simulink subsystem "PvtSubSys_VSM_ALL"  (R2020b)
settings: Solver=VariableStepAuto  StartTime=0.0  StopTime=10.0  RelTol=1e-3
values from neighbouring files (symbols this model uses):
  P_VSM_NOH_Act_Req = 0    [VSM_All.sldd]
  P_VSM_NOH_Swt_Req = 0    [VSM_All.sldd]
undefined symbols (not defined in the file or in its folder): ACC_STATE, HWA_STATE, LCK_STATE, P_VSM_ACCSOS_SW, P_VSM_AESSwtReq, P_VSM_CruiseFunUserInputMappingWays, P_VSM_ELKSwtReq, P_VSM_ESS_VehSwtReq, P_VSM_HWA_DMS_Enable, P_VSM_ICA_HandsOffSwtReq, P_VSM_IntelligentEvaSwtReq, P_VSM_ISLSwtReq, P_VSM_LCKSwtReq, P_VSM_LDWSwtReq, P_VSM_LKASwtReq, P_VSM_LSSSwtReq, P_VSM_PowerTrainConfig, P_VSM_SOSContinueTime, P_VSM_SOSSpdLimit, P_VSM_TSR_Dis_keep_SPL_Table, P_VSM_TSR_Dis_keep_SPLend, P_VSM_TSR_Dis_keep_TS_Table, P_VSM_TSR_Ena_SPLSupp_Table, P_VSM_TSR_Ena_TS_Table, P_VSM_TSR_SLIF_Speed_High, P_VSM_TSR_SLIF_Speed_Low, P_VSM_TSR_SLW_SnvtySwitch, P_VSM_TSR_SLW_Speed_Delta_disable, P_VSM_TSR_SLW_Speed_Delta_enable, P_VSM_TSR_SLW_Speed_High, P_VSM_TSR_SLW_Speed_Low, P_VSM_TSR_SLW_TrafEyeAvtiveDist, P_VSM_TSR_SLW_Warning_Time, P_VSM_TSR_SteerWheelAngle, P_VSM_TSR_SWS_speed_withDir, P_VSM_TSR_SWS_speed_woDir, P_VSM_TSRSwtReq, P_VSM_TSRWarnSwtReq, TJA_STATE, User_LC_ALCswt, User_LC_DrvConfirm, User_LC_DrvLCswt, User_LC_DrvOverride, User_LC_LeTurnNextLineReq, User_LC_RiTurnNextLineReq, User_LC_TurnMostLeLineReq, User_LC_TurnMostRiLineReq, User_LeTurnLmpOn, User_RiTurnLmpOn
libraries: simulink x51
(part 3 of 7)

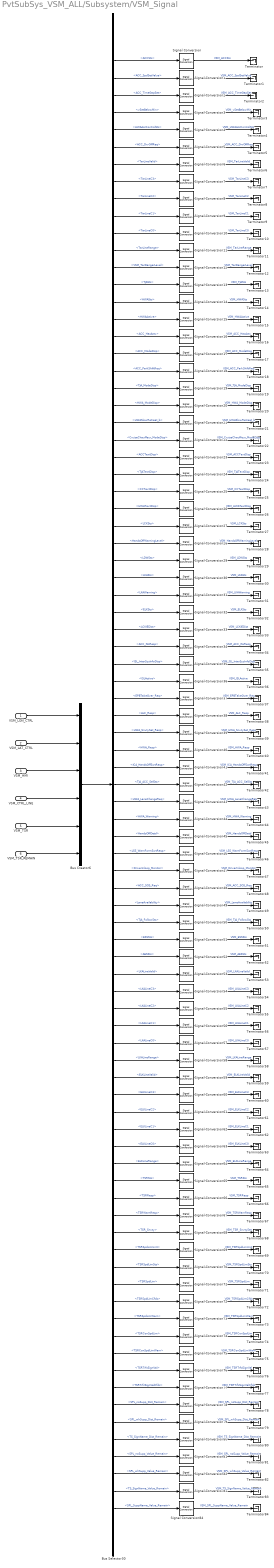
== system PvtSubSys_VSM_ALL/Subsystem/VSM_Signal ==
  VSM_LON_CTRL : Inport
  VSM_LAT_CTRL : Inport  Port=2
  VSM_HMI : Inport  Port=3
  VSM_CTRL_LINE : Inport  Port=4
  VSM_TSR : Inport  Port=5
  VSM_TSR_REMAIN : Inport  Port=6
  Bus Creator6 : BusCreator  Inputs=6
  Bus Selector30 : BusSelector  OutputSignals=VSM_LON_CTRL.ACCSts,VSM_LON_CTRL.ACC_SpdSetValue,VSM_LON_CTRL.ACC_TimeGapSet,VSM_LON_CTRL.vSetBelowMin,VSM_LON_CTRL.HWAAccControlSts,VSM_LON_CTRL.ACC_DrvOffReq,VSM_LAT_CTRL.TarLineValid,VSM_LAT_CTRL.TarLineC3,VSM_LAT_CTRL.TarLineC2,VSM_LAT_CTRL.TarLineC1,VSM_LAT_CTRL.TarLineC0,VSM_LAT_CTRL.TarLineRange,VSM_LAT_CTRL.VSM_TarDangerLevel,VSM_HMI.TJASts,VSM_HMI.HWASts,VSM_HMI.HWAActive,VSM_HMI.ACC_HazActv,VSM_HMI.ACC_ModeDisp,VSM_HMI.ACC_ParkShiftReq,VSM_HMI.TJA_ModeDisp,VSM_HMI.HWA_ModeDisp,VSM_HMI.HWASlowRetreat_b,VSM_HMI.CruiseChauffeur_ModeDisp,VSM_HMI.ACCTextDisp,VSM_HMI.TJATextDisp,VSM_HMI.CCTextDisp,VSM_HMI.HWATextDisp,VSM_HMI.LCKSts,VSM_HMI.HandsOffWarningLevel,VSM_HMI.LDWSts,VSM_HMI.LKASts,VSM_HMI.LKAWarning,VSM_HMI.ELKSts,VSM_HMI.LCKIEDist,VSM_HMI.ACC_ISLResp,VSM_HMI.ISL_InterSysInfoDisp,VSM_HMI.ISLActive,VSM_HMI.EPBTakeOver_Req,VSM_HMI.ALC_Resp,VSM_HMI.HWA_SnvtySet_Resp,VSM_HMI.HWA_Resp,VSM_HMI.ICA_HandsOffSwtResp,VSM_HMI.TJA_ACC_SelSts,VSM_HMI.HWA_LaneChangeReq,VSM_HMI.HWA_Warning,VSM_HMI.HandsOffDetd,VSM_HMI.LSS_WarnFormSwtResp,VSM_HMI.DriverInloop_Monitor,VSM_HMI.ACC_SOS_Req,VSM_HMI.LaneAvailability,VSM_HMI.TJA_FollowSts,VSM_HMI.ESSSts,VSM_HMI.AESSts,VSM_CTRL_LINE.LKALineValid,VSM_CTRL_LINE.LKALineC3,VSM_CTRL_LINE.LKALineC2,VSM_CTRL_LINE.LKALineC1,VSM_CTRL_LINE.LKALineC0,VSM_CTRL_LINE.LKALineRange,VSM_CTRL_LINE.ELKLineValid,VSM_CTRL_LINE.ELKLineC3,VSM_CTRL_LINE.ELKLineC2,VSM_CTRL_LINE.ELKLineC1,VSM_CTRL_LINE.ELKLineC0,VSM_CTRL_LINE.ELKLineRange,VSM_TSR.TSRSts,VSM_TSR.TSRResp,VSM_TSR.TSRWarnResp,VSM_TSR.TSR_Snvty,VSM_TSR.TSRSpdLimUnit,VSM_TSR.TSRSpdLimSts,VSM_TSR.TSRSpdLim,VSM_TSR.TSRSpdLimCfdc,VSM_TSR.TSRSpdLimWarn,VSM_TSR.TSRConSpdLim,VSM_TSR.TSRConSpdLimWarn,VSM_TSR.TSRTrfcSignVal,VSM_TSR.TSRTrfcSignValCfdc,VSM_TSR_REMAIN.SPL_noSupp_Dist_Remain,VSM_TSR_REMAIN.SPL_whSupp_Dist_Remain,VSM_TSR_REMAIN.TS_SignName_Dist_Remain,VSM_TSR_REMAIN.SPL_noSupp_Value_Remain,VSM_TSR_REMAIN.SPL_whSupp_Value_Remain,VSM_TSR_REMAIN.TS_SignName_Value_Remain,VSM_TSR_REMAIN.SPL_SuppName_Value_Remain
  Signal Conversion{,1..84} (85 alike) : SignalConversion  OverrideOpt=off
  Terminator{,1..84} (85 alike) : Terminator
  wires:
  Signal Conversion84/1 -> Terminator84/1  "VSM_SPL_SuppName_Value_Remain"
  Bus Selector30/85 -> Signal Conversion84/1  "<SPL_SuppName_Value_Remain>"
  Bus Selector30/84 -> Signal Conversion83/1  "<TS_SignName_Value_Remain>"
  Signal Conversion83/1 -> Terminator83/1  "VSM_TS_SignName_Value_Remain"
  Signal Conversion82/1 -> Terminator82/1  "VSM_SPL_whSupp_Value_Remain"
  Bus Selector30/83 -> Signal Conversion82/1  "<SPL_whSupp_Value_Remain>"
  Bus Selector30/82 -> Signal Conversion81/1  "<SPL_noSupp_Value_Remain>"
  Signal Conversion81/1 -> Terminator81/1  "VSM_SPL_noSupp_Value_Remain"
  Signal Conversion80/1 -> Terminator80/1  "VSM_TS_SignName_Dist_Remain"
  Bus Selector30/81 -> Signal Conversion80/1  "<TS_SignName_Dist_Remain>"
  Bus Selector30/80 -> Signal Conversion79/1  "<SPL_whSupp_Dist_Remain>"
  Signal Conversion79/1 -> Terminator79/1  "VSM_SPL_whSupp_Dist_Remain"
  Signal Conversion78/1 -> Terminator78/1  "VSM_SPL_noSupp_Dist_Remain"
  Bus Selector30/79 -> Signal Conversion78/1  "<SPL_noSupp_Dist_Remain>"
  Bus Selector30/78 -> Signal Conversion77/1  "<TSRTrfcSignValCfdc>"
  Signal Conversion77/1 -> Terminator77/1  "VSM_TSRTrfcSignValCfdc"
  Signal Conversion76/1 -> Terminator76/1  "VSM_TSRTrfcSignVal"
  Bus Selector30/77 -> Signal Conversion76/1  "<TSRTrfcSignVal>"
  Bus Selector30/76 -> Signal Conversion75/1  "<TSRConSpdLimWarn>"
  Signal Conversion75/1 -> Terminator75/1  "VSM_TSRConSpdLimWarn"
  Signal Conversion74/1 -> Terminator74/1  "VSM_TSRConSpdLim"
  Bus Selector30/75 -> Signal Conversion74/1  "<TSRConSpdLim>"
  Bus Selector30/74 -> Signal Conversion73/1  "<TSRSpdLimWarn>"
  Signal Conversion73/1 -> Terminator73/1  "VSM_TSRSpdLimWarn"
  Signal Conversion72/1 -> Terminator72/1  "VSM_TSRSpdLimCfdc"
  Bus Selector30/73 -> Signal Conversion72/1  "<TSRSpdLimCfdc>"
  Bus Selector30/72 -> Signal Conversion71/1  "<TSRSpdLim>"
  Signal Conversion71/1 -> Terminator71/1  "VSM_TSRSpdLim"
  Signal Conversion70/1 -> Terminator70/1  "VSM_TSRSpdLimSts"
  Bus Selector30/71 -> Signal Conversion70/1  "<TSRSpdLimSts>"
  Bus Selector30/70 -> Signal Conversion69/1  "<TSRSpdLimUnit>"
  Signal Conversion69/1 -> Terminator69/1  "VSM_TSRSpdLimUnit"
  Signal Conversion68/1 -> Terminator68/1  "VSM_TSR_SnvtySet"
  Bus Selector30/69 -> Signal Conversion68/1  "<TSR_Snvty>"
  Bus Selector30/68 -> Signal Conversion67/1  "<TSRWarnResp>"
  Signal Conversion67/1 -> Terminator67/1  "VSM_TSRWarnResp"
  Signal Conversion66/1 -> Terminator66/1  "VSM_TSRResp"
  Bus Selector30/67 -> Signal Conversion66/1  "<TSRResp>"
  Bus Selector30/66 -> Signal Conversion65/1  "<TSRSts>"
  Signal Conversion65/1 -> Terminator65/1  "VSM_TSRSts"
  Signal Conversion64/1 -> Terminator64/1  "VSM_ELKLineRange"
  Bus Selector30/65 -> Signal Conversion64/1  "<ELKLineRange>"
  Bus Selector30/64 -> Signal Conversion63/1  "<ELKLineC0>"
  Signal Conversion63/1 -> Terminator63/1  "VSM_ELKLineC0"
  Signal Conversion62/1 -> Terminator62/1  "VSM_ELKLineC1"
  Bus Selector30/63 -> Signal Conversion62/1  "<ELKLineC1>"
  Bus Selector30/62 -> Signal Conversion61/1  "<ELKLineC2>"
  Signal Conversion61/1 -> Terminator61/1  "VSM_ELKLineC2"
  Signal Conversion60/1 -> Terminator60/1  "VSM_ELKLineC3"
  Bus Selector30/61 -> Signal Conversion60/1  "<ELKLineC3>"
  Bus Selector30/60 -> Signal Conversion59/1  "<ELKLineValid>"
  Signal Conversion59/1 -> Terminator59/1  "VSM_ELKLineValid"
  Signal Conversion58/1 -> Terminator58/1  "VSM_LKALineRange"
  Bus Selector30/59 -> Signal Conversion58/1  "<LKALineRange>"
  Bus Selector30/58 -> Signal Conversion57/1  "<LKALineC0>"
  Signal Conversion57/1 -> Terminator57/1  "VSM_LKALineC0"
  Signal Conversion56/1 -> Terminator56/1  "VSM_LKALineC1"
  Bus Selector30/57 -> Signal Conversion56/1  "<LKALineC1>"
  Bus Selector30/56 -> Signal Conversion55/1  "<LKALineC2>"
  Signal Conversion55/1 -> Terminator55/1  "VSM_LKALineC2"
  Signal Conversion54/1 -> Terminator54/1  "VSM_LKALineC3"
  Bus Selector30/55 -> Signal Conversion54/1  "<LKALineC3>"
  Bus Selector30/54 -> Signal Conversion53/1  "<LKALineValid>"
  Signal Conversion53/1 -> Terminator53/1  "VSM_LKALineValid"
  Signal Conversion52/1 -> Terminator52/1  "VSM_AESSts"
  Bus Selector30/53 -> Signal Conversion52/1  "<AESSts>"
  Bus Selector30/52 -> Signal Conversion51/1  "<ESSSts>"
  Signal Conversion51/1 -> Terminator51/1  "VSM_ESSSts"
  Signal Conversion50/1 -> Terminator50/1  "VSM_TJA_FollowSts"
  Bus Selector30/51 -> Signal Conversion50/1  "<TJA_FollowSts>"
  Bus Selector30/50 -> Signal Conversion49/1  "<LaneAvailability>"
  Signal Conversion49/1 -> Terminator49/1  "VSM_LaneAvailability"
  Signal Conversion48/1 -> Terminator48/1  "VSM_ACC_SOS_Req"
  Bus Selector30/49 -> Signal Conversion48/1  "<ACC_SOS_Req>"
  Bus Selector30/48 -> Signal Conversion47/1  "<DriverInloop_Monitor>"
  Signal Conversion47/1 -> Terminator47/1  "VSM_DriverInloop_Monitor"
  Signal Conversion46/1 -> Terminator46/1  "VSM_LSS_WarnFormSwtResp"
  Bus Selector30/47 -> Signal Conversion46/1  "<LSS_WarnFormSwtResp>"
  Bus Selector30/46 -> Signal Conversion45/1  "<HandsOffDetd>"
  Signal Conversion45/1 -> Terminator45/1  "VSM_HandsOffDetd"
  Signal Conversion44/1 -> Terminator44/1  "VSM_HWA_Warning"
  Bus Selector30/45 -> Signal Conversion44/1  "<HWA_Warning>"
  Bus Selector30/44 -> Signal Conversion43/1  "<HWA_LaneChangeReq>"
  Signal Conversion43/1 -> Terminator43/1  "VSM_HWA_LaneChangeReq"
  Signal Conversion42/1 -> Terminator42/1  "VSM_TJA_ACC_SelSts"
  Bus Selector30/43 -> Signal Conversion42/1  "<TJA_ACC_SelSts>"
  Bus Selector30/42 -> Signal Conversion41/1  "<ICA_HandsOffSwtResp>"
  Signal Conversion41/1 -> Terminator41/1  "VSM_ICA_HandsOffSwtResp"
  Signal Conversion40/1 -> Terminator40/1  "VSM_HWA_Resp"
  Bus Selector30/41 -> Signal Conversion40/1  "<HWA_Resp>"
  Bus Selector30/40 -> Signal Conversion39/1  "<HWA_SnvtySet_Resp>"
  Signal Conversion39/1 -> Terminator39/1  "VSM_HWA_SnvtySet_Resp"
  Signal Conversion38/1 -> Terminator38/1  "VSM_ALC_Resp"
  Bus Selector30/39 -> Signal Conversion38/1  "<ALC_Resp>"
  Bus Selector30/38 -> Signal Conversion37/1  "<EPBTakeOver_Req>"
  Signal Conversion37/1 -> Terminator37/1  "VSM_EPBTakeOver_Req"
  Signal Conversion36/1 -> Terminator36/1  "VSM_ISLActive"
  Bus Selector30/37 -> Signal Conversion36/1  "<ISLActive>"
  Bus Selector30/36 -> Signal Conversion35/1  "<ISL_InterSysInfoDisp>"
  Signal Conversion35/1 -> Terminator35/1  "VSM_ISL_InterSysInfoDisp"
  Signal Conversion34/1 -> Terminator34/1  "VSM_ACC_ISLResp"
  Bus Selector30/35 -> Signal Conversion34/1  "<ACC_ISLResp>"
  Bus Selector30/34 -> Signal Conversion33/1  "<LCKIEDist>"
  Signal Conversion33/1 -> Terminator33/1  "VSM_LCKIEDist"
  Signal Conversion32/1 -> Terminator32/1  "VSM_ELKSts"
  Bus Selector30/33 -> Signal Conversion32/1  "<ELKSts>"
  Bus Selector30/32 -> Signal Conversion31/1  "<LKAWarning>"
  Signal Conversion31/1 -> Terminator31/1  "VSM_LKAWarning"
  Signal Conversion30/1 -> Terminator30/1  "VSM_LKASts"
  Bus Selector30/31 -> Signal Conversion30/1  "<LKASts>"
  Bus Selector30/30 -> Signal Conversion29/1  "<LDWSts>"
  Signal Conversion29/1 -> Terminator29/1  "VSM_LDWSts"
  Signal Conversion28/1 -> Terminator28/1  "VSM_HandsOffWarningLevel"
  Bus Selector30/29 -> Signal Conversion28/1  "<HandsOffWarningLevel>"
  Bus Selector30/28 -> Signal Conversion27/1  "<LCKSts>"
  Signal Conversion27/1 -> Terminator27/1  "VSM_LCKSts"
  Signal Conversion26/1 -> Terminator26/1  "VSM_HWATextDisp"
  Bus Selector30/27 -> Signal Conversion26/1  "<HWATextDisp>"
  Bus Selector30/26 -> Signal Conversion25/1  "<CCTextDisp>"
  Signal Conversion25/1 -> Terminator25/1  "VSM_CCTextDisp"
  Signal Conversion24/1 -> Terminator24/1  "VSM_TJATextDisp"
  Bus Selector30/25 -> Signal Conversion24/1  "<TJATextDisp>"
  Bus Selector30/24 -> Signal Conversion23/1  "<ACCTextDisp>"
  Signal Conversion23/1 -> Terminator23/1  "VSM_ACCTextDisp"
  Signal Conversion22/1 -> Terminator22/1  "VSM_CruiseChauffeur_ModeDisp"
  Bus Selector30/23 -> Signal Conversion22/1  "<CruiseChauffeur_ModeDisp>"
  Bus Selector30/22 -> Signal Conversion21/1  "<HWASlowRetreat_b>"
  Signal Conversion21/1 -> Terminator21/1  "VSM_HWASlowRetreat_b"
  Signal Conversion20/1 -> Terminator20/1  "VSM_HWA_ModeDisp"
  Bus Selector30/21 -> Signal Conversion20/1  "<HWA_ModeDisp>"
  Bus Selector30/20 -> Signal Conversion19/1  "<TJA_ModeDisp>"
  Signal Conversion19/1 -> Terminator19/1  "VSM_TJA_ModeDisp"
  Signal Conversion18/1 -> Terminator18/1  "VSM_ACC_ParkShiftReq"
  Bus Selector30/19 -> Signal Conversion18/1  "<ACC_ParkShiftReq>"
  Bus Selector30/18 -> Signal Conversion17/1  "<ACC_ModeDisp>"
  Signal Conversion17/1 -> Terminator17/1  "VSM_ACC_ModeDisp"
  Signal Conversion16/1 -> Terminator16/1  "VSM_ACC_HazActv"
  Bus Selector30/17 -> Signal Conversion16/1  "<ACC_HazActv>"
  Bus Selector30/16 -> Signal Conversion15/1  "<HWAActive>"
  Signal Conversion15/1 -> Terminator15/1  "VSM_HWAActive"
  Signal Conversion14/1 -> Terminator14/1  "VSM_HWASts"
  Bus Selector30/15 -> Signal Conversion14/1  "<HWASts>"
  Bus Selector30/14 -> Signal Conversion13/1  "<TJASts>"
  Signal Conversion13/1 -> Terminator13/1  "VSM_TJASts"
  Signal Conversion12/1 -> Terminator12/1  "VSM_TarDangerLevel"
  Bus Selector30/13 -> Signal Conversion12/1  "<VSM_TarDangerLevel>"
  Bus Selector30/12 -> Signal Conversion11/1  "<TarLineRange>"
  Signal Conversion11/1 -> Terminator11/1  "VSM_TarLineRange"
  Signal Conversion10/1 -> Terminator10/1  "VSM_TarLineC0"
  Bus Selector30/11 -> Signal Conversion10/1  "<TarLineC0>"
  Bus Selector30/10 -> Signal Conversion9/1  "<TarLineC1>"
  Signal Conversion9/1 -> Terminator9/1  "VSM_TarLineC1"
  Signal Conversion8/1 -> Terminator8/1  "VSM_TarLineC2"
  Bus Selector30/9 -> Signal Conversion8/1  "<TarLineC2>"
  Bus Selector30/8 -> Signal Conversion7/1  "<TarLineC3>"
  Signal Conversion7/1 -> Terminator7/1  "VSM_TarLineC3"
  Signal Conversion6/1 -> Terminator6/1  "VSM_TarLineValid"
  Bus Selector30/7 -> Signal Conversion6/1  "<TarLineValid>"
  Bus Selector30/6 -> Signal Conversion5/1  "<ACC_DrvOffReq>"
  Signal Conversion5/1 -> Terminator5/1  "VSM_ACC_DrvOffReq"
  Signal Conversion4/1 -> Terminator4/1  "VSM_HWAAccControlSts"
  Bus Selector30/5 -> Signal Conversion4/1  "<HWAAccControlSts>"
  Bus Selector30/4 -> Signal Conversion3/1  "<vSetBelowMin>"
  Signal Conversion3/1 -> Terminator3/1  "VSM_vSetBelowMin"
  Signal Conversion2/1 -> Terminator2/1  "VSM_ACC_TimeGapSet"
  Bus Selector30/3 -> Signal Conversion2/1  "<ACC_TimeGapSet>"
  Bus Selector30/2 -> Signal Conversion1/1  "<ACC_SpdSetValue>"
  Signal Conversion1/1 -> Terminator1/1  "VSM_ACC_SpdSetValue"
  Signal Conversion/1 -> Terminator/1  "VSM_ACCSts"
  VSM_CTRL_LINE/1 -> Bus Creator6/4
  VSM_LON_CTRL/1 -> Bus Creator6/1
  VSM_HMI/1 -> Bus Creator6/3
  VSM_TSR_REMAIN/1 -> Bus Creator6/6
  VSM_TSR/1 -> Bus Creator6/5
  VSM_LAT_CTRL/1 -> Bus Creator6/2
  Bus Selector30/1 -> Signal Conversion/1  "<ACCSts>"
  Bus Creator6/1 -> Bus Selector30/1

== system PvtSubSys_VSM_ALL/Subsystem/StateManage/Cruise ==
  LCKStateInfo : Inport
  ALC : Inport  Port=2
  UserOperation : Inport  Port=3
  VehConfig : Inport  Port=4
  Diag : Inport  Port=5
  TSR_Info : Inport  Port=6
  DriverSts : Inport  Port=7
  EHR_Input : Inport  Port=8
  ACC_P0 : Inport  Port=9
  VehicleSts : Inport  Port=10
  AD_CAN : Inport  Port=11
  Target_Line : Inport  Port=12
  ESSState : Inport  Port=13
  PilotSts : Inport  Port=14
  HODinfo : Inport  Port=15
  PLAN_NOH_SetSpdAdjReq : Inport  Port=16
  PLAN_NOH_SetSpdAdjVal : Inport  Port=17
  LSM_PilotNohExitDist : Inport  Port=18
  TimeGapInit : Inport  Port=19
  IB_BrkPedalAppld : Inport  Port=20
  ConfigiBooster : Inport  Port=21
  Bus Creator : BusCreator  Inputs=2
  Bus Creator1 : BusCreator  Inputs=5
  Bus Creator13 : BusCreator  Inputs=31
  Bus Selector : BusSelector  OutputSignals=axvRefMs2,vxvRefMs,DriveOffConditionFulfilled,AEB_TgtDecel_Req,Longctrl_Decel_ReqValue
  Bus Selector1 : BusSelector  OutputSignals=LSM_HWA.DoubleLineLost_b,LSM_HWA.HWALineValid,LSM_TJA_ICA.TJALineValid
  Bus Selector42 : BusSelector  OutputSignals=LCK_State,TJA_LCKState
  Bus Selector5 : BusSelector  OutputSignals=ACC_Error,HWA_Error,TJA_ICA_Error
  Bus Selector55 : BusSelector  OutputSignals=targetExistP0,dxP0
  Bus Selector6 : BusSelector  OutputSignals=VehConfigHWA,VehConfigTJA,VehConfigACC,VehConfigiACC
  Cruise : Subsystem
  Signal Conversion : SignalConversion  OverrideOpt=off
  Signal Conversion1 : SignalConversion  OverrideOpt=off
  tt2 : Ground
  EDR_Longitude_HWAExit : Outport
  UOMSysFeedBack : Outport  Port=2
  EDR_ACCDataClct : Outport  Port=3
  HWAStateInfo : Outport  Port=4
  HWA_TurnLightReq : Outport  Port=5
  ACC_TimeGapSetHMI : Outport  Port=6
  wires:
  ConfigiBooster/1 -> Cruise/35(ConfigiBooster)
  IB_BrkPedalAppld/1 -> Cruise/34(IB_BrkPedalAppld)
  TimeGapInit/1 -> Cruise/33(TimeGapInit)
  Cruise/42(ACC_TimeGapSetHMI) -> ACC_TimeGapSetHMI/1
  Bus Selector5/3 -> Cruise/3("\tTJAError")  "<TJA_ICA_Error>"
  Signal Conversion1/1 -> Cruise/20(TJALineValid)
  Bus Selector1/3 -> Signal Conversion1/1  "<TJALineValid>"
  Cruise/31(HWAParkShiftReq) -> Bus Creator13/31
  Cruise/30(Signal_NOH_DistToExit) -> Bus Creator13/30
  Cruise/29(Signal_NOH_SysInfoDisplay) -> Bus Creator13/29
  Cruise/28(Signal_NOH_Sts) -> Bus Creator13/28
  LSM_PilotNohExitDist/1 -> Cruise/32(LSM_PilotNohExitDist)
  Cruise/27(Signal_DriverOffDisp) -> Bus Creator13/27
  Bus Selector55/2 -> Cruise/10(<dxP0>)  "<dxP0>"
  PLAN_NOH_SetSpdAdjVal/1 -> Cruise/31(PLAN_NOH_SetSpdAdjVal)
  PLAN_NOH_SetSpdAdjReq/1 -> Cruise/30(PLAN_NOH_SetSpdAdjReq)
  Cruise/40(HWA_TurnLightReq) -> HWA_TurnLightReq/1
  Bus Selector42/2 -> Cruise/17(TJA_LCKState)  "<TJA_LCKState>"
  Bus Creator1/1 -> EDR_ACCDataClct/1
  Cruise/39(TJADataClct_ConNotStsf) -> Bus Creator1/5  "TJADataClct_ConNotStsf"
  Cruise/38(ACCDataClct_DriverSteerACCExit) -> Bus Creator1/4
  Cruise/37(ACCDataClct_DriverBrakeACCExit) -> Bus Creator1/3
  Cruise/36(ACCDataClct_OverrideACCExit) -> Bus Creator1/2
  Cruise/35(ACCDataClct_ConNotStsf) -> Bus Creator1/1
  tt2/1 -> Cruise/8(ObjFailure_b)
  DriverSts/1 -> Cruise/22(DriverSts)
  Cruise/4(Signal_ACC_TimeGapSet) -> Bus Creator13/4
  Cruise/7(Signal_ACC_ModDisp) -> Bus Creator13/7
  Bus Selector42/1 -> Cruise/16(LCK_State)  "<LCK_State>"
  Cruise/8(Signal_TJA_ACC_SelSts) -> Bus Creator13/8
  Cruise/13(Signal_CruiseChauffer_Sts) -> Bus Creator13/13
  Bus Selector1/2 -> Signal Conversion/1  "<HWALineValid>"
  Cruise/16(Signal_CCTextDisp) -> Bus Creator13/16
  Bus Selector1/1 -> Cruise/18(DoubleLineLost_b)  "<DoubleLineLost_b>"
  Cruise/2(Signal_ACC_SpdSetValue) -> Bus Creator13/2
  Bus Selector/2 -> Cruise/12(VxvRef_ms)  "<vxvRefMs>"
  Cruise/17(HWASts) -> Bus Creator13/17
  Cruise/22(ISL_Resp) -> Bus Creator13/22
  Cruise/21(Signal_HWAModeDisp) -> Bus Creator13/21
  Cruise/19(HWAActive) -> Bus Creator13/19
  Cruise/23(ISL_InterSysInfoDisp) -> Bus Creator13/23
  Cruise/5(Signal_ACC_DrvOFF_Req) -> Bus Creator13/5
  Bus Selector/4 -> Cruise/14(AEB_Trigger)  "<AEB_TgtDecel_Req>"
  Cruise/18(TJASts) -> Bus Creator13/18
  Bus Selector5/1 -> Cruise/1(ACCError)  "<ACC_Error>"
  Bus Selector/3 -> Cruise/13(DriveOffConditonFulfilled_b)  "<DriveOffConditionFulfilled>"
  VehicleSts/1 -> Bus Selector/1
  Cruise/11(ACCParkShiftReq) -> Bus Creator13/11
  Bus Creator13/1 -> HWAStateInfo/1  "HWAStateInfo"
  Cruise/15(Signal_TJATextDisp) -> Bus Creator13/15
  Cruise/14(Signal_ACCTextDisp) -> Bus Creator13/14
  Bus Selector5/2 -> Cruise/2(HWAError)  "<HWA_Error>"
  Bus Selector55/1 -> Cruise/9(TargetExist_b)  "<targetExistP0>"
  Cruise/6(vSetBelowMin) -> Bus Creator13/6
  Cruise/10(Signal_ACC_ModeSts) -> Bus Creator13/10
  Cruise/3(Signal_ACC_HazActv) -> Bus Creator13/3
  Cruise/12(Signal_TJA_ModeSts) -> Bus Creator13/12
  Cruise/20(HWAWarningLevel) -> Bus Creator13/20
  Cruise/24(ISLActive) -> Bus Creator13/24
  EHR_Input/1 -> Cruise/29(EHR_Input)
  LCKStateInfo/1 -> Bus Selector42/1
  Diag/1 -> Bus Selector5/1
  Target_Line/1 -> Bus Selector1/1
  ACC_P0/1 -> Bus Selector55/1
  TSR_Info/1 -> Cruise/23(TSR_output)
  VehConfig/1 -> Bus Selector6/1
  Bus Selector6/1 -> Cruise/4(VehConfigHWA)  "<VehConfigHWA>"
  Bus Selector6/2 -> Cruise/5(VehConfigTJA)  "<VehConfigTJA>"
  Bus Selector6/3 -> Cruise/6(VehConfigACC)  "<VehConfigACC>"
  Bus Selector6/4 -> Cruise/7(VehConfigiACC)  "<VehConfigiACC>"
  Bus Selector/1 -> Cruise/11(axvRefMs2)  "<axvRefMs2>"
  Bus Selector/5 -> Cruise/15(Longctrl_Decel_ReqValue)  "<Longctrl_Decel_ReqValue>"
  AD_CAN/1 -> Cruise/21(AD_CAN)
  Cruise/9(TJA_ON) -> Bus Creator13/9
  Cruise/25(SetSpeedKmh) -> Bus Creator13/25
  Cruise/1(HWA_LaneChangeReq) -> Bus Creator13/1
  Cruise/32(EDR_DriverBrakeHWAExit) -> Bus Creator/1
  Cruise/33(EDR_OverrideHWAExit) -> Bus Creator/2
  Bus Creator/1 -> EDR_Longitude_HWAExit/1
  HODinfo/1 -> Cruise/25(HODinfo)
  Cruise/26(Signal_HWATextDisp) -> Bus Creator13/26
  ALC/1 -> Cruise/26(ALC)
  Signal Conversion/1 -> Cruise/19(HWALineValid)
  Cruise/34(UOMSysFeedBack) -> UOMSysFeedBack/1
  UserOperation/1 -> Cruise/24(DirverOperation)
  ESSState/1 -> Cruise/27(VSM_ESSState)
  PilotSts/1 -> Cruise/28(PilotSts)

== system PvtSubSys_VSM_ALL/Subsystem/StateManage/EDR_HWAExit ==
  HWAActive_b : Inport
  <EDR_DriverBrakeHWAExit> : Inport  Port=2
  <EDR_OverrideHWAExit> : Inport  Port=3
  <VSM_LCK_Con_SteerAngleSpd_Active2Ready> : Inport  Port=4
  <VSM_LCK_Con_OverRide_Active2Ready> : Inport  Port=5
  <VSM_LCK_Con_SteerWheelAngle_Active2Ready> : Inport  Port=6
  <VSM_LCK_Con_DriverInput_Active2Ready> : Inport  Port=7
  Bus Creator : BusCreator  Inputs=3
  Logical Operator16 : Logic  AllPortsSameDT=off  OutDataTypeStr=boolean
  Logical Operator17 : Logic  AllPortsSameDT=off  OutDataTypeStr=boolean
  Logical Operator18 : Logic  Operator=OR  Inputs=4  AllPortsSameDT=off  OutDataTypeStr=boolean
  Logical Operator19 : Logic  AllPortsSameDT=off  OutDataTypeStr=boolean
  MATLAB Function1 : MATLAB Function  TreatAsAtomicUnit=on
  MATLAB Function2 : MATLAB Function  TreatAsAtomicUnit=on
  MATLAB Function3 : MATLAB Function  TreatAsAtomicUnit=on
  Unit Delay : UnitDelay  SampleTime=-1  HasFrameUpgradeWarning=on
  Unit Delay1 : UnitDelay  SampleTime=-1  HasFrameUpgradeWarning=on
  Unit Delay2 : UnitDelay  SampleTime=-1  HasFrameUpgradeWarning=on
  HWA_DATA : Outport
  wires:
  Bus Creator/1 -> HWA_DATA/1
  MATLAB Function1/2(Counter) -> Unit Delay1/1
  Unit Delay/1 -> MATLAB Function2/2(CounterK1)
  HWAActive_b/1 -> Logical Operator19/1, Logical Operator17/1, Logical Operator16/1
  MATLAB Function2/2(Counter) -> Unit Delay/1
  Logical Operator18/1 -> Logical Operator19/2
  Unit Delay1/1 -> MATLAB Function1/2(CounterK1)
  Logical Operator17/1 -> MATLAB Function1/1(HWAExit_b)
  <EDR_OverrideHWAExit>/1 -> Logical Operator17/2
  Unit Delay2/1 -> MATLAB Function3/2(CounterK1)
  Logical Operator19/1 -> MATLAB Function3/1(HWAExit_b)
  MATLAB Function3/2(Counter) -> Unit Delay2/1
  <VSM_LCK_Con_SteerWheelAngle_Active2Ready>/1 -> Logical Operator18/3
  Logical Operator16/1 -> MATLAB Function2/1(HWAExit_b)
  <EDR_DriverBrakeHWAExit>/1 -> Logical Operator16/2
  MATLAB Function1/1(y) -> Bus Creator/2  "HWADATAClct_OverrideHWAExit"
  <VSM_LCK_Con_SteerAngleSpd_Active2Ready>/1 -> Logical Operator18/1
  <VSM_LCK_Con_DriverInput_Active2Ready>/1 -> Logical Operator18/4
  <VSM_LCK_Con_OverRide_Active2Ready>/1 -> Logical Operator18/2
  MATLAB Function2/1(y) -> Bus Creator/1  "HWADATAClct_DriverBrakeHWAExit"
  MATLAB Function3/1(y) -> Bus Creator/3  "HWADATAClct_DriverSteerHWAExit"

== system PvtSubSys_VSM_ALL/Subsystem/StateManage/ESS ==
  ESS_SideViewSts : Inport
  VehicleSts : Inport  Port=2
  AD_CAN : Inport  Port=3
  Target_Line : Inport  Port=4
  AEB_OBJ : Inport  Port=5
  Dia : Inport  Port=6
  VehConfig : Inport  Port=7
  Bus Creator : BusCreator  Inputs=25
  Bus Creator1 : BusCreator  Inputs=2
  Bus Creator2 : BusCreator  Inputs=3
  Bus Selector : BusSelector  OutputSignals=AEB_PedTrig,AEB_VehTrig,Inter_FCW_Warn
  Bus Selector1 : BusSelector  OutputSignals=VehSpd,VDCActv,PTCActv,BTCActv,ABSActv,EPS_DrvInpTrqVal_HighReslolution,SteerWheelSpd,AccelPedlPosnDiagc,VehLatAccel,EPS_LKATorqOvrlDlvd,SteerWheelSpdSign,FrntWiprSwtSts,HighBeamSts,LowBeamSts,ESPFuncOffSts,DrvDoorSts,PassengerDoorSts,DrvSBR,VehLgtAccel,MSRActv,ESS_PedSwtReq,ESS_VehSwtReq,EPS_LKATrqOvlDlvdSts,ESP_MasterCylBrkPress,SteerWheelAngSign
  Bus Selector2 : BusSelector  OutputSignals=LSM_ESS,LSM_HWA.RoadWidth
  Bus Selector3 : BusSelector  OutputSignals=ESS_Error
  Bus Selector4 : BusSelector  OutputSignals=VehConfigESS
  ESS : Subsystem  ReferencedSubsystem=PvtSubSys_VSM_ESS
  VSM_ESSState : Outport
  ESS_DATA : Outport  Port=2
  wires:
  Bus Selector1/24 -> Bus Creator/24  "<ESP_MasterCylBrkPress>"
  Bus Selector2/2 -> ESS/5  "<RoadWidth>"
  Bus Selector1/23 -> Bus Creator/23  "<EPS_LKATrqOvlDlvdSts>"
  Bus Selector4/1 -> ESS/8  "<VehConfigESS>"
  Bus Selector3/1 -> ESS/7  "<ESS_Error>"
  VehConfig/1 -> Bus Selector4/1
  Dia/1 -> Bus Selector3/1
  Bus Selector2/1 -> ESS/4  "<LSM_ESS>"
  Bus Creator2/1 -> ESS/2
  Bus Selector/3 -> Bus Creator2/3  "<Inter_FCW_Warn>"
  Bus Selector/2 -> Bus Creator2/2  "<AEB_VehTrig>"
  Bus Selector/1 -> Bus Creator2/1  "<AEB_PedTrig>"
  Bus Creator1/1 -> ESS_DATA/1
  ESS/3 -> Bus Creator1/2
  ESS/2 -> Bus Creator1/1
  Bus Creator/1 -> ESS/3
  Bus Selector1/22 -> Bus Creator/22  "<ESS_VehSwtReq>"
  Bus Selector1/21 -> Bus Creator/21  "<ESS_PedSwtReq>"
  Bus Selector1/20 -> Bus Creator/20  "<MSRActv>"
  Bus Selector1/19 -> Bus Creator/19  "<VehLgtAccel>"
  Bus Selector1/18 -> Bus Creator/18  "<DrvSBR>"
  Bus Selector1/17 -> Bus Creator/17  "<PassengerDoorSts>"
  Bus Selector1/16 -> Bus Creator/16  "<DrvDoorSts>"
  Bus Selector1/15 -> Bus Creator/15  "<ESPFuncOffSts>"
  Bus Selector1/9 -> Bus Creator/9  "<VehLatAccel>"
  Bus Selector1/8 -> Bus Creator/8  "<AccelPedlPosnDiagc>"
  Bus Selector1/7 -> Bus Creator/7  "<SteerWheelSpd>"
  Bus Selector1/6 -> Bus Creator/6  "<EPS_DrvInpTrqVal_HighReslolution>"
  Bus Selector1/5 -> Bus Creator/5  "<ABSActv>"
  Bus Selector1/4 -> Bus Creator/4  "<BTCActv>"
  Bus Selector1/3 -> Bus Creator/3  "<PTCActv>"
  Bus Selector1/2 -> Bus Creator/2  "<VDCActv>"
  Bus Selector1/1 -> Bus Creator/1  "<VehSpd>"
  Bus Selector1/11 -> Bus Creator/11  "<SteerWheelSpdSign>"
  Bus Selector1/12 -> Bus Creator/12  "<FrntWiprSwtSts>"
  Bus Selector1/14 -> Bus Creator/14  "<LowBeamSts>"
  Bus Selector1/10 -> Bus Creator/10  "<EPS_LKATorqOvrlDlvd>"
  Bus Selector1/13 -> Bus Creator/13  "<HighBeamSts>"
  AD_CAN/1 -> Bus Selector1/1
  ESS/1 -> VSM_ESSState/1
  ESS_SideViewSts/1 -> ESS/1
  Target_Line/1 -> Bus Selector2/1
  AEB_OBJ/1 -> ESS/6
  VehicleSts/1 -> Bus Selector/1
  Bus Selector1/25 -> Bus Creator/25  "<SteerWheelAngSign>"

== system PvtSubSys_VSM_ALL/Subsystem/StateManage/Enlong2s1 ==
  note: 拨打E_Call 持续时间
  VSM_HWA_ParkShiftReq : Inport
  TJASts : Inport  Port=2
  vehspd : Inport  Port=3
  AND : Logic  AllPortsSameDT=off  OutDataTypeStr=boolean
  AND1 : Logic  AllPortsSameDT=off  OutDataTypeStr=boolean
  AND2 : Logic  AllPortsSameDT=off  OutDataTypeStr=boolean
  Add : Sum
  Chart : Stateflow chart  TreatAsAtomicUnit=on
  Compare To Constant : simulink/Logic and Bit Operations/Compare To Constant  relop=>  const=0.5  OutDataTypeStr=boolean
  Compare To Constant1 : simulink/Logic and Bit Operations/Compare To Constant  relop===  const=1  OutDataTypeStr=boolean
  Compare To Constant2 : simulink/Logic and Bit Operations/Compare To Constant  relop===  const=0  OutDataTypeStr=boolean
  Compare To Constant25 : simulink/Logic and Bit Operations/Compare To Constant  relop===  const=TJA_STATE.TJA_SafeStop  OutDataTypeStr=boolean
  Compare To Constant26 : simulink/Logic and Bit Operations/Compare To Constant  relop===  const=TJA_STATE.TJA_Active  OutDataTypeStr=boolean
  Compare To Constant8 : simulink/Logic and Bit Operations/Compare To Constant  relop===  const=TJA_STATE.TJA_SlowRetreat  OutDataTypeStr=boolean
  Constant : Constant  Value=1.3
  Constant1 : Constant  Value=P_VSM_SOSSpdLimit
  Gain : Gain  Gain=1.03
  MATLAB Function : MATLAB Function  TreatAsAtomicUnit=on
  OR : Logic  Operator=OR  AllPortsSameDT=off  OutDataTypeStr=boolean
  SignalRising : Subsystem
  Switch20 : Switch  Criteria=u2 ~= 0
  Time : Constant  Value=P_VSM_SOSContinueTime  OutDataTypeStr=uint16
  Unit Delay{,2..4} (4 alike) : UnitDelay  SampleTime=-1  HasFrameUpgradeWarning=on
  Unit Delay1 : UnitDelay  InitialCondition=TJA_STATE.TJA_Active  SampleTime=-1  HasFrameUpgradeWarning=on
  Out1 : Outport
  wires:
  AND2/1 -> Chart/4(ACCSOS)
  Compare To Constant2/1 -> AND2/2
  Compare To Constant1/1 -> AND2/1
  Unit Delay4/1 -> Compare To Constant1/1
  Chart/1(SW) -> AND/1
  Constant1/1 -> Chart/1(P_VSM_SOSSpd_SW)
  Add/1 -> Chart/2(vehspd)
  AND1/1 -> Chart/3(state)
  Compare To Constant25/1 -> AND1/2
  OR/1 -> AND1/1
  Compare To Constant26/1 -> OR/2
  Compare To Constant8/1 -> OR/1
  Constant/1 -> Add/2
  Gain/1 -> Add/1
  vehspd/1 -> Gain/1
  AND/1 -> Out1/1
  Unit Delay1/1 -> Compare To Constant8/1, Compare To Constant26/1
  TJASts/1 -> Compare To Constant25/1, Unit Delay1/1
  Time/1 -> MATLAB Function/3(Num)
  Switch20/1 -> AND/2, Unit Delay2/1, Compare To Constant2/1, Unit Delay4/1
  Unit Delay2/1 -> Switch20/1
  Unit Delay3/1 -> MATLAB Function/2(X)
  Compare To Constant/1 -> Switch20/2
  MATLAB Function/1(Cnt) -> Compare To Constant/1, Unit Delay/1
  Unit Delay/1 -> MATLAB Function/1(CntK1)
  SignalRising/1(Out1) -> Unit Delay3/1
  VSM_HWA_ParkShiftReq/1 -> SignalRising/1(In1), Switch20/3

== system PvtSubSys_VSM_ALL/Subsystem/StateManage/HOD ==
  EPS_DrvInpTrqVal_HighReslolution : Inport
  HWAStateInfo : Inport  Port=2
  LatStateInfo : Inport  Port=3
  Bus Selector : BusSelector  OutputSignals=LCK_State,ELK_State,LKA_State
  Bus Selector1 : BusSelector  OutputSignals=TJASts,VSM_HWAActive
  Bus Selector4 : BusSelector  OutputSignals=EPS_DrvInpTrqVal_HighReslolution,VehStandstill
  Bus Creator : BusCreator  Inputs=2
  HOD : Subsystem  ReferencedSubsystem=PvtSubSys_VSM_HOD
  HODinfo : Outport
  wires:
  Bus Selector1/2 -> HOD/4  "<VSM_HWAActive>"
  LatStateInfo/1 -> Bus Selector/1
  HWAStateInfo/1 -> Bus Selector1/1
  Bus Selector/1 -> HOD/5  "<LCK_State>"
  Bus Selector/3 -> HOD/7  "<LKA_State>"
  Bus Selector/2 -> HOD/6  "<ELK_State>"
  Bus Selector1/1 -> HOD/3  "<TJASts>"
  Bus Creator/1 -> HODinfo/1  "HODinfo"
  EPS_DrvInpTrqVal_HighReslolution/1 -> Bus Selector4/1
  Bus Selector4/1 -> HOD/1  "<EPS_DrvInpTrqVal_HighReslolution>"
  HOD/2 -> Bus Creator/2
  HOD/1 -> Bus Creator/1
  Bus Selector4/2 -> HOD/2  "<VehStandstill>"

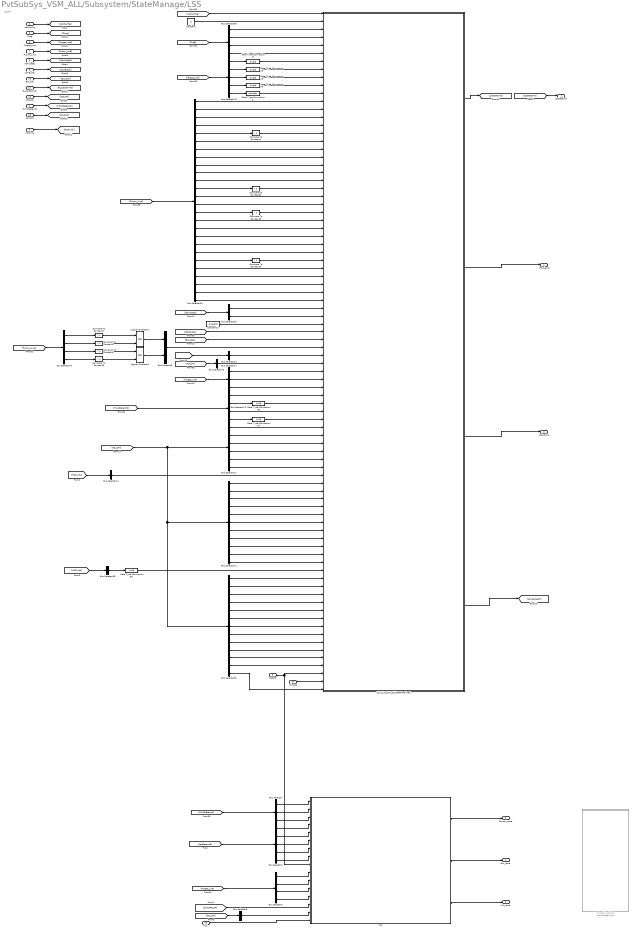
== system PvtSubSys_VSM_ALL/Subsystem/StateManage/LSS ==
  note: Signal
  HWAStateInfo : Inport
  VehConfig : Inport  Port=2
  Diag : Inport  Port=3
  HODinfo : Inport  Port=4
  ESSSts : Inport  Port=5
  Target_Line : Inport  Port=6
  Fusion_Line : Inport  Port=7
  VehicleSts : Inport  Port=8
  LCKIE_Obj : Inport  Port=9
  ELK_Obj : Inport  Port=10
  BusLatCtrlInfo : Inport  Port=11
  ACC_P0 : Inport  Port=12
  AD_CAN : Inport  Port=13
  PilotSts : Inport  Port=14
  ALC : Inport  Port=15
  Bus Creator15 : BusCreator  Inputs=2
  Bus Selector : BusSelector  OutputSignals=VSM_HWAActive,VSM_HWASts,TJASts
  Bus Selector1 : BusSelector  OutputSignals=ELK_State,LKA_State,LCKIE_State,LCK_State,LCKIE_Laneoffset
  Bus Selector11 : BusSelector  OutputSignals=VehSpd,VehYawRate,VDCActv,PTCActv,BTCActv,ABSActv
  Bus Selector12 : BusSelector  OutputSignals=SteerWheelAng,EPS_DrvInpTrqVal_HighReslolution,SteerWheelSpd,VehLatAccel,VehLgtAccel,ESP_MasterCylBrkPress,AccelPedlPosnDiagc,EPS_LKATrqOvlDlvdSts,CURRENT_GEAR,LTurnLmpSwtSts,RTurnLmpSwtSts
  Bus Selector13 : BusSelector  OutputSignals=epsTrqReqValue
  Bus Selector14 : BusSelector  OutputSignals=HandsOffDetd
  Bus Selector2 : BusSelector  OutputSignals=LSM_LCK,LSM_TJA_ICA,LSM_HWA,LSM_ESS
  Bus Selector3 : BusSelector  OutputSignals=HWA_SnvtySet
  Bus Selector34 : BusSelector  OutputSignals=RFM_LINE_L1.dC0V,RFM_LINE_L1.dC1V,RFM_LINE_L1.dC2V,RFM_LINE_L1.dC3V,RFM_LINE_L1.bIsLineExist,RFM_LINE_L1.dDisFront,RFM_LINE_L1.eLineType,RFM_LINE_R1.dC0V,RFM_LINE_R1.dC1V,RFM_LINE_R1.dC2V,RFM_LINE_R1.dC3V,RFM_LINE_R1.bIsLineExist,RFM_LINE_R1.dDisFront,RFM_LINE_R1.eLineType,RFM_LINEF_LB.bIsLineExist,RFM_LINEF_LB.dC0V,RFM_LINEF_LB.dC1V,RFM_LINEF_LB.dC2V,RFM_LINEF_LB.dC3V,RFM_LINEF_LB.dDisFront,RFM_LINEF_RB.bIsLineExist,RFM_LINEF_RB.dC0V,RFM_LINEF_RB.dC1V,RFM_LINEF_RB.dC2V,RFM_LINEF_RB.dC3V,RFM_LINEF_RB.dDisFront
  Bus Selector35 : BusSelector  OutputSignals=LKA_LCK_Error,LKA_LCK_Error,LDW_Error,ELK_Error
  Bus Selector36 : BusSelector  OutputSignals=FrntWiprSwtSts,HighBeamSts,LowBeamSts,RFogLmpSts_R_Pbox,FFogLmpSts_F_Pbox,LCKSwtReq,LKASwtReq,ELKSwtReq,LDWSwtReq,IntelligentEvaSwtReq,IFC_SnvtySet,LSSSwtReq,BrkPedalSts
  Bus Selector37 : BusSelector  OutputSignals=LSM_HWA.HWALineValid,LSM_TJA_ICA,LSM_LCK.LCKLineValid
  Bus Selector38 : BusSelector  OutputSignals=HandsOffWarnLevel
  Bus Selector39 : BusSelector  OutputSignals=vxvRefMs,kapTraj
  Bus Selector44 : BusSelector  OutputSignals=RFM_LINE_L1.bIsLineExist,RFM_LINE_R1.bIsLineExist,RFM_LINEF_LB.bIsLineExist,RFM_LINEF_RB.bIsLineExist
  Bus Selector72 : BusSelector  OutputSignals=targetExistP0
  Bus Selector73 : BusSelector  OutputSignals=VSM_HWAActive,TJASts,TJAOn,VSM_HWASts
  Bus Selector79 : BusSelector  OutputSignals=LSM_LCK.LCKLineC0,LSM_LCK.LCKLineC1,LSM_LCK.LCKLineC2,LSM_LCK.LCKLineC3,LSM_LCK.LCKLineValid
  Compare To Constant{1..8} (8 alike) : simulink/Logic and Bit Operations/Compare To Constant  relop=>  const=1  OutDataTypeStr=boolean
  Constant : Constant  Value=0
  Constant17 : Constant  Value=single(0)
  Data Type Conversion{27..30} (4 alike) : DataTypeConversion  OutDataTypeStr=single
  Data Type Conversion3 : DataTypeConversion  OutDataTypeStr=boolean
  Data Type Conversion66 : DataTypeConversion  OutDataTypeStr=uint8
  Data Type Conversion67 : DataTypeConversion  OutDataTypeStr=uint8
  Data Type Conversion69 : DataTypeConversion  OutDataTypeStr=uint8
  LCK_LKA_LDW_ELKStateMachine3 : Subsystem
  Logical Operator1 : Logic  Operator=OR  AllPortsSameDT=off  OutDataTypeStr=boolean
  Logical Operator2 : Logic  Operator=OR  AllPortsSameDT=off  OutDataTypeStr=boolean
  TLS : Subsystem  ReferencedSubsystem=PvtSubSys_VSM_TLS
  TargetLineSelect : Subsystem  Commented=on
  LatStateInfo : Outport
  IFC_Signal : Outport  Port=2
  Control_Lane : Outport  Port=3
  ELK_Lane : Outport  Port=4
  LKA_Lane : Outport  Port=5
  LSS_DATA : Outport  Port=6
  wires:
  ALC/1 -> TLS/16
  Bus Selector36/13 -> LCK_LKA_LDW_ELKStateMachine3/86(BrkPedalSts)  "<BrkPedalSts>"
  Bus Selector3/1 -> TLS/15  "<HWA_SnvtySet>"
  [AD_CAN] -> Bus Selector3/1
  PilotSts/1 -> LCK_LKA_LDW_ELKStateMachine3/85(PilotSts)
  [LaneARe_SP] -> TLS/14
  LCK_LKA_LDW_ELKStateMachine3/4(LaneARe_SP) -> [LaneARe_SP]
  LCK_LKA_LDW_ELKStateMachine3/3(LSS_DATA) -> LSS_DATA/1
  Bus Selector2/3 -> TLS/12  "<LSM_HWA>"
  Bus Selector2/2 -> TLS/11  "<LSM_TJA_ICA>"
  Bus Selector2/1 -> TLS/10  "<LSM_LCK>"
  Bus Selector2/4 -> TLS/13  "<LSM_ESS>"
  Bus Selector1/5 -> TLS/8  "<LCKIE_Laneoffset>"
  Bus Selector1/4 -> TLS/7  "<LCK_State>"
  Bus Selector1/3 -> TLS/6  "<LCKIE_State>"
  Bus Selector1/2 -> TLS/5  "<LKA_State>"
  Bus Selector1/1 -> TLS/4  "<ELK_State>"
  Bus Selector/3 -> TLS/3  "<TJASts>"
  Bus Selector/2 -> TLS/2  "<VSM_HWASts>"
  Bus Selector/1 -> TLS/1  "<VSM_HWAActive>"
  Bus Selector12/11 -> LCK_LKA_LDW_ELKStateMachine3/70(canBCMRightTurnSWSts)  "<RTurnLmpSwtSts>"
  Bus Selector11/1 -> LCK_LKA_LDW_ELKStateMachine3/53(canABSVehicleSpd)  "<VehSpd>"
  Bus Selector12/6 -> LCK_LKA_LDW_ELKStateMachine3/65(canESP_MasterCylindBrakePress)  "<ESP_MasterCylBrkPress>"
  Bus Selector36/6 -> LCK_LKA_LDW_ELKStateMachine3/77(canHUTLCKSwtReq)  "<LCKSwtReq>"
  [Fusion_Line] -> Bus Selector44/1
  Bus Selector34/4 -> LCK_LKA_LDW_ELKStateMachine3/15(laneLeftA3)  "<dC3V>"
  Bus Selector36/5 -> LCK_LKA_LDW_ELKStateMachine3/76(canBCMFrontFogLmpSts)  "<FFogLmpSts_F_Pbox>"
  Bus Selector36/7 -> LCK_LKA_LDW_ELKStateMachine3/78(canHUTLKASwtReq)  "<LKASwtReq>"
  Bus Selector36/1 -> LCK_LKA_LDW_ELKStateMachine3/72(canBCMWiperSwitchSts)  "<FrntWiprSwtSts>"
  [LCKIE_Obj] -> LCK_LKA_LDW_ELKStateMachine3/41(LCKIEBus)
  [AD_CAN] -> Bus Selector11/1, Bus Selector36/1, Bus Selector12/1
  Bus Selector34/11 -> LCK_LKA_LDW_ELKStateMachine3/22(laneRightA3)  "<dC3V>"
  [BusLatCtrlInfo] -> Bus Selector13/1
  Bus Selector12/1 -> LCK_LKA_LDW_ELKStateMachine3/60(canSASSteerWheelAngle)  "<SteerWheelAng>"
  Logical Operator2/1 -> Bus Creator15/2  "VisEdgeUpdate"
  Bus Selector36/3 -> LCK_LKA_LDW_ELKStateMachine3/74(canBCMLowBeamSts)  "<LowBeamSts>"
  Bus Selector12/5 -> LCK_LKA_LDW_ELKStateMachine3/64(LongitudeAcc)  "<VehLgtAccel>"
  Bus Selector11/2 -> LCK_LKA_LDW_ELKStateMachine3/54(canABMVehDynYawRate)  "<VehYawRate>"
  Compare To Constant6/1 -> LCK_LKA_LDW_ELKStateMachine3/32(F_RBbIsLineExist)
  Compare To Constant5/1 -> LCK_LKA_LDW_ELKStateMachine3/23(laneRightValid)
  Bus Selector35/1 -> LCK_LKA_LDW_ELKStateMachine3/3(LCKError)  "<LKA_LCK_Error>"
  Bus Selector12/3 -> LCK_LKA_LDW_ELKStateMachine3/62(canSASSteerWheelSpd)  "<SteerWheelSpd>"
  LCK_LKA_LDW_ELKStateMachine3/2(IFC_Signal) -> IFC_Signal/1
  Bus Selector79/2 -> Data Type Conversion28/1  "<LCKLineC1>"
  [Diag] -> Bus Selector35/1
  Bus Selector12/2 -> LCK_LKA_LDW_ELKStateMachine3/61(canEPS_DriverInputTrqValue)  "<EPS_DrvInpTrqVal_HighReslolution>"
  Compare To Constant7/1 -> Logical Operator1/1
  Bus Selector37/3 -> LCK_LKA_LDW_ELKStateMachine3/48(LCKLineValid)  "<LCKLineValid>"
  Bus Selector34/10 -> LCK_LKA_LDW_ELKStateMachine3/21(laneRightA2)  "<dC2V>"
  Logical Operator1/1 -> Bus Creator15/1  "VisLaneUpdate"
  Bus Selector11/5 -> LCK_LKA_LDW_ELKStateMachine3/57(canESPBTCActive)  "<BTCActv>"
  Bus Creator15/1 -> LCK_LKA_LDW_ELKStateMachine3/43(LIneEdgeUpdate)
  Bus Selector36/8 -> LCK_LKA_LDW_ELKStateMachine3/79(canHUTELKSwtReq)  "<ELKSwtReq>"
  Bus Selector12/9 -> LCK_LKA_LDW_ELKStateMachine3/68(CURRENT_GEAR)  "<CURRENT_GEAR>"
  Bus Selector36/11 -> LCK_LKA_LDW_ELKStateMachine3/82(IFC_SnvtySet)  "<IFC_SnvtySet>"
  Bus Selector12/4 -> LCK_LKA_LDW_ELKStateMachine3/63(canABMLateralAcce)  "<VehLatAccel>"
  Bus Selector36/9 -> LCK_LKA_LDW_ELKStateMachine3/80(canHUTLDWSwtReq)  "<LDWSwtReq>"
  Bus Selector11/3 -> LCK_LKA_LDW_ELKStateMachine3/55(canESPVDCActive)  "<VDCActv>"
  Bus Selector36/10 -> LCK_LKA_LDW_ELKStateMachine3/81(IntelligentEvaSwtReq)  "<IntelligentEvaSwtReq>"
  Bus Selector34/7 -> LCK_LKA_LDW_ELKStateMachine3/18(laneLeftType)  "<eLineType>"
  Bus Selector34/6 -> LCK_LKA_LDW_ELKStateMachine3/17(laneLeftRange)  "<dDisFront>"
  LCK_LKA_LDW_ELKStateMachine3/1(LCS_OutPut) -> [LatStateInfo]
  Bus Selector36/4 -> LCK_LKA_LDW_ELKStateMachine3/75(canBCMRearFogLmpSts)  "<RFogLmpSts_R_Pbox>"
  [ACC_P0] -> Bus Selector72/1
  Compare To Constant2/1 -> Logical Operator2/1
  Bus Selector11/6 -> LCK_LKA_LDW_ELKStateMachine3/58(canABSABSActive)  "<ABSActv>"
  Bus Selector12/7 -> LCK_LKA_LDW_ELKStateMachine3/66(canECMAccrPedlPosnDiagc)  "<AccelPedlPosnDiagc>"
  [VehConfig] -> LCK_LKA_LDW_ELKStateMachine3/1(VehConfig)
  Bus Selector11/4 -> LCK_LKA_LDW_ELKStateMachine3/56(canESPPTCActive)  "<PTCActv>"
  Bus Selector34/9 -> LCK_LKA_LDW_ELKStateMachine3/20(laneRightA1)  "<dC1V>"
  Bus Selector34/12 -> Compare To Constant5/1  "<bIsLineExist>"
  Bus Selector12/8 -> LCK_LKA_LDW_ELKStateMachine3/67(canEPS_LKATrqOvlDlvdSts)  "<EPS_LKATrqOvlDlvdSts>"
  Bus Selector44/2 -> Compare To Constant1/1  "<bIsLineExist>"
  Bus Selector35/4 -> LCK_LKA_LDW_ELKStateMachine3/6(ELKError)  "<ELK_Error>"
  Constant/1 -> LCK_LKA_LDW_ELKStateMachine3/2(IFC_FailSafe)
  Compare To Constant3/1 -> Logical Operator2/2
  Compare To Constant4/1 -> LCK_LKA_LDW_ELKStateMachine3/16(laneLeftValid)
  Bus Selector44/4 -> Compare To Constant3/1  "<bIsLineExist>"
  [HODinfo] -> Bus Selector38/1
  Compare To Constant8/1 -> LCK_LKA_LDW_ELKStateMachine3/26(F_LBbIsLineExist)
  [HODinfo] -> Bus Selector14/1
  Bus Selector44/1 -> Compare To Constant7/1  "<bIsLineExist>"
  Bus Selector12/10 -> LCK_LKA_LDW_ELKStateMachine3/69(canBCMLeftTurnSWSts)  "<LTurnLmpSwtSts>"
  [HWAStateInfo] -> Bus Selector73/1
  Bus Selector79/3 -> Data Type Conversion29/1  "<LCKLineC2>"
  Bus Selector36/2 -> LCK_LKA_LDW_ELKStateMachine3/73(canBCMHighBeamSts)  "<HighBeamSts>"
  Bus Selector34/20 -> LCK_LKA_LDW_ELKStateMachine3/31(RELeft_Range)  "<dDisFront>"
  Bus Selector34/1 -> LCK_LKA_LDW_ELKStateMachine3/12(laneLeftA0)  "<dC0V>"
  Bus Selector34/3 -> LCK_LKA_LDW_ELKStateMachine3/14(laneLeftA2)  "<dC2V>"
  [VehicleSts] -> Bus Selector39/1
  Bus Selector35/3 -> LCK_LKA_LDW_ELKStateMachine3/5(LDWError)  "<LDW_Error>"
  [Target_Line] -> Bus Selector37/1
  Bus Selector79/5 -> Data Type Conversion3/1  "<LCKLineValid>"
  Bus Selector34/5 -> Compare To Constant4/1  "<bIsLineExist>"
  Bus Selector34/13 -> LCK_LKA_LDW_ELKStateMachine3/24(laneRightRange)  "<dDisFront>"
  Bus Selector34/8 -> LCK_LKA_LDW_ELKStateMachine3/19(laneRightA0)  "<dC0V>"
  Bus Selector34/2 -> LCK_LKA_LDW_ELKStateMachine3/13(laneLeftA1)  "<dC1V>"
  Bus Selector39/2 -> LCK_LKA_LDW_ELKStateMachine3/39(EVI_Kap)  "<kapTraj>"
  Bus Selector34/14 -> LCK_LKA_LDW_ELKStateMachine3/25(laneRightType)  "<eLineType>"
  Bus Selector39/1 -> LCK_LKA_LDW_ELKStateMachine3/38(EVI_VehicleSpd_ms)  "<vxvRefMs>"
  [Target_Line] -> Bus Selector79/1
  Bus Selector72/1 -> LCK_LKA_LDW_ELKStateMachine3/45(targetExistP0)  "<targetExistP0>"
  [Fusion_Line] -> Bus Selector34/1
  Bus Selector44/3 -> Compare To Constant2/1  "<bIsLineExist>"
  Compare To Constant1/1 -> Logical Operator1/2
  Bus Selector37/1 -> LCK_LKA_LDW_ELKStateMachine3/46(HWALineValid)  "<HWALineValid>"
  Bus Selector37/2 -> LCK_LKA_LDW_ELKStateMachine3/47(TJALineValid)  "<LSM_TJA_ICA>"
  Constant17/1 -> LCK_LKA_LDW_ELKStateMachine3/40(EVI_alpSideSlipAngle)
  [ELK_Obj] -> LCK_LKA_LDW_ELKStateMachine3/42(ELK_ObjBus)
  Bus Selector79/4 -> Data Type Conversion30/1  "<LCKLineC3>"
  Bus Selector35/2 -> LCK_LKA_LDW_ELKStateMachine3/4(LKAError)  "<LKA_LCK_Error>"
  Bus Selector13/1 -> LCK_LKA_LDW_ELKStateMachine3/44(TrqK1)  "<epsTrqReqValue>"
  Bus Selector79/1 -> Data Type Conversion27/1  "<LCKLineC0>"
  [Target_Line] -> Bus Selector2/1
  TLS/3 -> LKA_Lane/1
  TLS/2 -> ELK_Lane/1
  TLS/1 -> Control_Lane/1
  ESSSts/1 -> TLS/9, LCK_LKA_LDW_ELKStateMachine3/84(ESSSts)
  VehConfig/1 -> [VehConfig]
  Diag/1 -> [Diag]
  Target_Line/1 -> [Target_Line]
  Fusion_Line/1 -> [Fusion_Line]
  VehicleSts/1 -> [VehicleSts]
  LCKIE_Obj/1 -> [LCKIE_Obj]
  ELK_Obj/1 -> [ELK_Obj]
  BusLatCtrlInfo/1 -> [BusLatCtrlInfo]
  ACC_P0/1 -> [ACC_P0]
  HWAStateInfo/1 -> [HWAStateInfo]
  AD_CAN/1 -> [AD_CAN]
  [LatStateInfo] -> LatStateInfo/1
  [HWAStateInfo] -> Bus Selector/1
  [LatStateInfo] -> Bus Selector1/1
  Bus Selector14/1 -> LCK_LKA_LDW_ELKStateMachine3/59(HandsOffDetect)  "<HandsOffDetd>"
  Bus Selector73/1 -> LCK_LKA_LDW_ELKStateMachine3/49(HWAActive)  "<VSM_HWAActive>"
  Bus Selector73/2 -> Data Type Conversion66/1  "<TJASts>"
  Bus Selector73/3 -> LCK_LKA_LDW_ELKStateMachine3/51(TJAOn)  "<TJAOn>"
  Bus Selector73/4 -> Data Type Conversion67/1  "<VSM_HWASts>"
  Bus Selector38/1 -> Data Type Conversion69/1  "<HandsOffWarnLevel>"
  Data Type Conversion3/1 -> LCK_LKA_LDW_ELKStateMachine3/11(LCKLane_Valid)
  Data Type Conversion27/1 -> LCK_LKA_LDW_ELKStateMachine3/7(LCKLane_A0)
  Data Type Conversion28/1 -> LCK_LKA_LDW_ELKStateMachine3/8(LCKLane_A1)
  Data Type Conversion29/1 -> LCK_LKA_LDW_ELKStateMachine3/9(LCKLane_A2)
  Data Type Conversion30/1 -> LCK_LKA_LDW_ELKStateMachine3/10(LCKLane_A3)
  Data Type Conversion66/1 -> LCK_LKA_LDW_ELKStateMachine3/50(TJASts)
  Data Type Conversion67/1 -> LCK_LKA_LDW_ELKStateMachine3/52(HWASts)
  Data Type Conversion69/1 -> LCK_LKA_LDW_ELKStateMachine3/71(HandsOffWarnLevel)
  HODinfo/1 -> [HODinfo]
  Bus Selector34/22 -> LCK_LKA_LDW_ELKStateMachine3/33(F_RBdC0V)  "<dC0V>"
  Bus Selector34/23 -> LCK_LKA_LDW_ELKStateMachine3/34(F_RBdC1V)  "<dC1V>"
  Bus Selector34/24 -> LCK_LKA_LDW_ELKStateMachine3/35(F_RBdC2V)  "<dC2V>"
  Bus Selector34/25 -> LCK_LKA_LDW_ELKStateMachine3/36(F_RBdC3V)  "<dC3V>"
  Bus Selector34/21 -> Compare To Constant6/1  "<bIsLineExist>"
  Bus Selector34/26 -> LCK_LKA_LDW_ELKStateMachine3/37(RERight_Range)  "<dDisFront>"
  Bus Selector34/15 -> Compare To Constant8/1  "<bIsLineExist>"
  Bus Selector34/16 -> LCK_LKA_LDW_ELKStateMachine3/27(F_LBdC0V)  "<dC0V>"
  Bus Selector34/17 -> LCK_LKA_LDW_ELKStateMachine3/28(F_LBdC1V)  "<dC1V>"
  Bus Selector34/18 -> LCK_LKA_LDW_ELKStateMachine3/29(F_LBdC2V)  "<dC2V>"
  Bus Selector34/19 -> LCK_LKA_LDW_ELKStateMachine3/30(F_LBdC3V)  "<dC3V>"
  Bus Selector36/12 -> LCK_LKA_LDW_ELKStateMachine3/83(LSSSwtReq)  "<LSSSwtReq>"

== system PvtSubSys_VSM_ALL/Subsystem/StateManage/TSR ==
  VehConfig : Inport
  Diag : Inport  Port=2
  ISL_Actice : Inport  Port=3
  RF_input : Inport  Port=4
  AD_CAN : Inport  Port=5
  VSM_TSR_Init : Inport  Port=6
  Bus Creator : BusCreator  Inputs=14
  Bus Selector1 : BusSelector  OutputSignals=TSRSwtReq,TSRWarnSwtReq,TSR_SnvtySet,SteerWheelAng,SteerWheelAngSign,VehSpd,IP_VehSpdUnit,RTurnLmpSwtSts,LTurnLmpSwtSts,VehYawRate,FFogLmpSts_F_Pbox,RFogLmpSts_R_Pbox,WindshldWiprActvSts,ACAmbTemp
  Bus Selector7 : BusSelector  OutputSignals=ISL_Active
  Bus Selector8 : BusSelector  OutputSignals=TSR_Error
  Bus Selector9 : BusSelector  OutputSignals=VehConfigTSR
  TSR : Subsystem  ReferencedSubsystem=PvtSubSys_VSM_TSR
  TSR_output : Outport
  wires:
  Bus Creator/1 -> TSR/5  "TSR_ADCAN"
  Bus Selector1/1 -> Bus Creator/1  "<TSRSwtReq>"
  Bus Selector1/14 -> Bus Creator/14  "<ACAmbTemp>"
  Bus Selector1/2 -> Bus Creator/2  "<TSRWarnSwtReq>"
  Bus Selector1/13 -> Bus Creator/13  "<WindshldWiprActvSts>"
  Bus Selector1/3 -> Bus Creator/3  "<TSR_SnvtySet>"
  Bus Selector1/12 -> Bus Creator/12  "<RFogLmpSts_R_Pbox>"
  Bus Selector1/4 -> Bus Creator/4  "<SteerWheelAng>"
  Bus Selector1/11 -> Bus Creator/11  "<FFogLmpSts_F_Pbox>"
  Bus Selector1/5 -> Bus Creator/5  "<SteerWheelAngSign>"
  Bus Selector1/10 -> Bus Creator/10  "<VehYawRate>"
  Bus Selector1/6 -> Bus Creator/6  "<VehSpd>"
  Bus Selector1/9 -> Bus Creator/9  "<LTurnLmpSwtSts>"
  Bus Selector1/7 -> Bus Creator/7  "<IP_VehSpdUnit>"
  Bus Selector1/8 -> Bus Creator/8  "<RTurnLmpSwtSts>"
  VehConfig/1 -> Bus Selector9/1
  Diag/1 -> Bus Selector8/1
  TSR/1 -> TSR_output/1
  Bus Selector7/1 -> TSR/3  "<ISL_Active>"
  Bus Selector8/1 -> TSR/2  "<TSR_Error>"
  RF_input/1 -> TSR/4
  Bus Selector9/1 -> TSR/1  "<VehConfigTSR>"
  VSM_TSR_Init/1 -> TSR/6
  ISL_Actice/1 -> Bus Selector7/1
  AD_CAN/1 -> Bus Selector1/1
